simulink model "VVI_proof_of_concept"  (R2020a)
settings: Solver=FixedStepAuto  StartTime=0.0  StopTime=10.0  FixedStep=1e-3  RelTol=1e-3  EnableMultiTasking=on
libraries: frdmk64flib x1
settings Model: EnablePacing=on  PacingRate=0.010000  ExtModeTrigDuration=5  Creator=Ethan  LastModifiedBy=Ethan
settings OptimizationCC: EnhancedBackFolding=on  PassReuseOutputArgsAs=Individual arguments  ZeroExternalMemoryAtStartup=off  ZeroInternalMemoryAtStartup=off  MaxStackSize=64  OptimizeBlockOrder=speed  DifferentSizesBufferReuse=on  OptimizationCustomize=off  EfficientTunableParamExpr=on
settings DebuggingCC: ParameterTunabilityLossMsg=error
settings HardwareCC: ProdBitPerPointer=32  ProdBitPerSizeT=32  ProdBitPerPtrDiffT=32  ProdLargestAtomicInteger=Long  ProdLargestAtomicFloat=Double  ProdWordSize=32  ProdHWDeviceType=ARM Compatible->ARM Cortex
settings SFSimCC: MATLABDynamicMemAlloc=off
settings RTWCC: SystemTargetFile=ert.tlc  HardwareBoard=NXP FRDM-K64F  TemplateMakefile=ert_default_tmf  Toolchain=GNU Tools for ARM Embedded Processors
settings CodeAppCC: ForceParamTrailComments=on  IgnoreCustomStorageClasses=off  OperatorAnnotations=on  SimulinkDataObjDesc=on  SFDataObjDesc=on  InsertBlockDesc=on

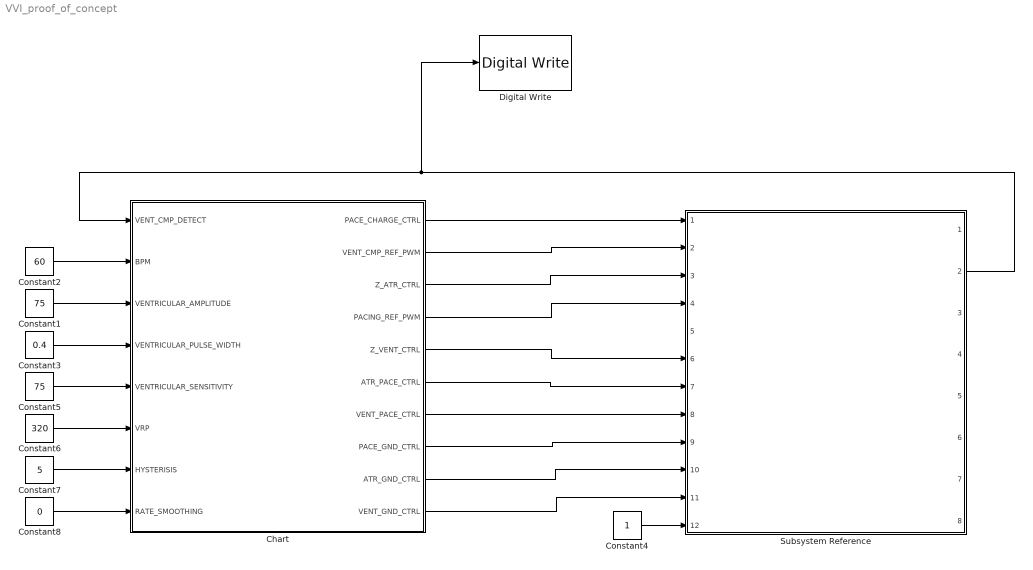
== system VVI_proof_of_concept ==
  Chart : Stateflow chart  TreatAsAtomicUnit=on
      settings: PortSchema="{\"entries\":[{\"content\":{\"sides\":[{\"content\":{\"connectorIds\":[\"In8\",\"In1\",\"In2\",\"In3\",\"In4\",\"In5\",\"In6\",\"In7\"]},\"type\":\"ConnectorPlacement.EquallySpacedRectSide\",\"uuid\":\"b678de6f-9e61-4024-a0aa-5bf6d03f3d0b\"},{\"content\":{\"connectorIds\":[\"Out3\",\"Out10\",\"Out8\",\"Out5\",\"Out9\",\"Out2\",\"Out7\",\"Out4\",\"Out1\",\"Out6\"],\"side\":\"RIGHT\"},\"type\":\"ConnectorPlacement.EquallySpacedRectSide\",\"uuid\":\"4cd0faad-dd9d-4a56-81c5-44f7dd4bee31\"},{\"content\":{\"connectorIds\":[],\"side\":\"TOP\"},\"type\":\"ConnectorPlacement.EquallySpacedRectSide\",\"uuid\":\"a9bc4227-6f84-42c8-b827-a378e14304fe\"}]},\"type\":\"ConnectorPlacement.EquallySpacedConnector\",\"uuid\":\"ee3b07ee-2423-4f21-89d4-53b7a563517d\"}],\"packageUris\":[\"http://schema.mathworks.com/mf0/Connector/19700101\"],\"version\":\"1.0\"}"
  Constant1 : Constant  Value=75
  Constant2 : Constant  Value=60
  Constant3 : Constant  Value=0.4
  Constant4 : Constant
  Constant5 : Constant  Value=75
  Constant6 : Constant  Value=320
  Constant7 : Constant  Value=5
  Constant8 : Constant  Value=0
  Digital Write : frdmk64flib/Digital Write  Whichpin=BLUE_LED
  Subsystem Reference : Subsystem  ReferencedSubsystem=k64f_subsystem
  wires:
  Constant2/1 -> Chart/1(BPM)
  Constant1/1 -> Chart/2(VENTRICULAR_AMPLITUDE)
  Constant3/1 -> Chart/3(VENTRICULAR_PULSE_WIDTH)
  Constant4/1 -> Subsystem Reference/12
  Constant5/1 -> Chart/4(VENTRICULAR_SENSITIVITY)
  Chart/9(Z_VENT_CTRL) -> Subsystem Reference/6
  Chart/5(PACING_REF_PWM) -> Subsystem Reference/4
  Chart/8(Z_ATR_CTRL) -> Subsystem Reference/3
  Chart/3(PACE_CHARGE_CTRL) -> Subsystem Reference/1
  Chart/2(ATR_PACE_CTRL) -> Subsystem Reference/7
  Chart/7(VENT_PACE_CTRL) -> Subsystem Reference/8
  Chart/4(PACE_GND_CTRL) -> Subsystem Reference/9
  Chart/1(ATR_GND_CTRL) -> Subsystem Reference/10
  Chart/6(VENT_GND_CTRL) -> Subsystem Reference/11
  Constant6/1 -> Chart/5(VRP)
  Constant7/1 -> Chart/6(HYSTERISIS)
  Constant8/1 -> Chart/7(RATE_SMOOTHING)
  Subsystem Reference/2 -> Chart/8(VENT_CMP_DETECT), Digital Write/1
  Chart/10(VENT_CMP_REF_PWM) -> Subsystem Reference/2

== stateflow chart VVI_proof_of_concept/Chart ==
  state hold
    entry:
  state INIT
    entry:
    VENT_CMP_REF_PWM = VENTRICULAR_SENSITIVITY;
    PACING_REF_PWM = VENTRICULAR_AMPLITUDE;
    ATR_GND_CTRL = 0;
    ATR_PACE_CTRL = 0;
    Z_ATR_CTRL = 0;
    Z_VENT_CTRL = 0;
    PACE_GND_CTRL = 1;
    last_pulse_natural = false;
  state PULSE_SET_NATURAL
    entry:
    last_pulse_natural = true;
  state PULSE_SET_ARTIFICIAL
    entry:
    last_pulse_natural = false;
  state PULSE_ATR
    entry:
    PACE_CHARGE_CTRL = 0;
    VENT_GND_CTRL = 0;
    VENT_PACE_CTRL = 1;
  state CHARGE
    entry:
    VENT_PACE_CTRL = 0;
    PACE_CHARGE_CTRL = 1;
  state DISCHARGE
    entry:
    VENT_PACE_CTRL = 0;
    VENT_GND_CTRL = 1;
  hold -> PULSE_SET_ARTIFICIAL [order 3] : after(60000/BPM-VENTRICULAR_PULSE_WIDTH-VRP, msec)[ last_pulse_natural == false || HYSTERISIS == 0]
  CHARGE -> hold : after(VRP, msec)
  hold -> PULSE_SET_ARTIFICIAL [order 2] : after(60000/(BPM-HYSTERISIS)-VENTRICULAR_PULSE_WIDTH-VRP, msec)[ last_pulse_natural == true && HYSTERISIS > 0]
  hold -> PULSE_SET_NATURAL [order 1] : [VENT_CMP_DETECT == 1]
  (default) -> INIT
  PULSE_SET_ARTIFICIAL -> PULSE_ATR
  PULSE_SET_NATURAL -> CHARGE
  INIT -> CHARGE
  DISCHARGE -> CHARGE
  PULSE_ATR -> DISCHARGE : after(VENTRICULAR_PULSE_WIDTH, msec)
  data: ATR_GND_CTRL output; ATR_PACE_CTRL output; PACE_CHARGE_CTRL output; PACE_GND_CTRL output; PACING_REF_PWM output; VENT_GND_CTRL output; VENT_PACE_CTRL output; Z_ATR_CTRL output; Z_VENT_CTRL output; BPM input; VENTRICULAR_AMPLITUDE input; VENTRICULAR_PULSE_WIDTH input; VENTRICULAR_SENSITIVITY input; VRP input; HYSTERISIS input; RATE_SMOOTHING input; VENT_CMP_REF_PWM output; VENT_CMP_DETECT input; last_pulse_natural local
